simulink model "vehicle_dynamic_dis"  (R2022b)
settings: Solver=VariableStepAuto  StartTime=0.0  StopTime=30  RelTol=1e-3
values from neighbouring files (symbols this model uses):
  A_dis = V_DIS.A    [vehicle_lateral_control_LMIs_3states_auto.m]
  B_dis = V_DIS.B    [vehicle_lateral_control_LMIs_3states_auto.m]
  C_dis = V_DIS.C    [vehicle_lateral_control_LMIs_3states_auto.m]
  D_dis = V_DIS.D    [vehicle_lateral_control_LMIs_3states_auto.m]
  K_gain = K_lmi    [vehicle_lateral_control_LMIs_3states_auto.m]
  Ts = 0.01    [vehicle_lateral_control_LMIs_3states_auto.m]
  vx = 14    [vehicle_lateral_control_LMIs_3states_auto.m]
libraries: cstblocks x1
settings Model: Creator=phatdo  LastModifiedBy=phatdo
settings DataIOCC: ReturnWorkspaceOutputs=off

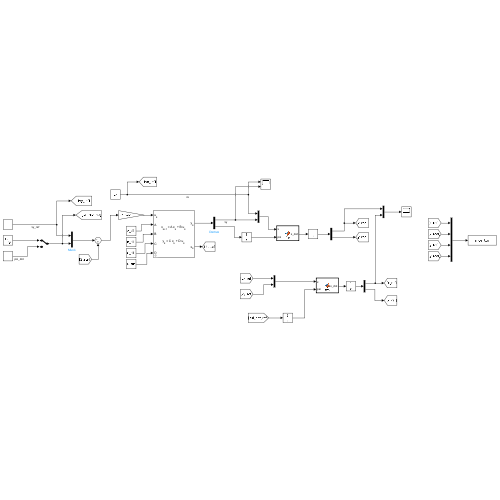
[thumbnail: Simulink's stored preview of the top-level diagram]
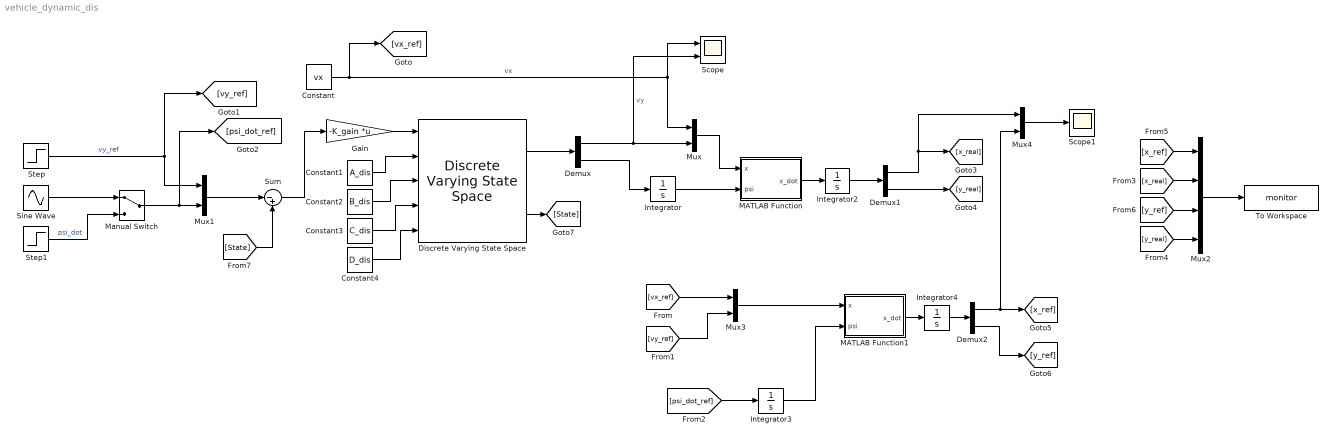
== system vehicle_dynamic_dis ==
  Constant : Constant  Value=vx
  Constant1 : Constant  Value=A_dis
  Constant2 : Constant  Value=B_dis
  Constant3 : Constant  Value=C_dis
  Constant4 : Constant  Value=D_dis
  Demux : Demux  Outputs=2
  Demux1 : Demux  Outputs=2
  Demux2 : Demux  Outputs=2
  Discrete Varying State Space : cstblocks/Linear Parameter Varying/Discrete Varying State Space  x0=0  Ts=Ts  OutputX=on  OutputDX=off
  Gain : Gain  Gain=-K_gain  Multiplication=Matrix(K*u) (u vector)
  Integrator{,2..4} (4 alike) : Integrator
  MATLAB Function : MATLAB Function  TreatAsAtomicUnit=on
  MATLAB Function1 : MATLAB Function  TreatAsAtomicUnit=on
  Manual Switch : ManualSwitch
  Mux{,1,3..4} (4 alike) : Mux  Inputs=2
  Mux2 : Mux
  Scope : Scope  NumInputPorts=2
  Scope1 : Scope
  Sine Wave : Sin  SampleTime=Ts
  Step : Step  Time=0  After=0  SampleTime=Ts
  Step1 : Step  Time=0  After=0.5  SampleTime=Ts
  Sum : Sum  Inputs=|-+
  To Workspace : ToWorkspace  VariableName=monitor  SaveFormat=Timeseries  SampleTime=-1
  wires:
  Discrete Varying State Space/1 -> Demux/1
  Constant/1 -> [vx_ref], Scope/1, Mux/1  "vx"
  Demux/1 -> Scope/2, Mux/2  "vy"
  Mux/1 -> MATLAB Function/1(x)
  Demux/2 -> Integrator/1
  Integrator/1 -> MATLAB Function/2(psi)
  MATLAB Function/1(x_dot) -> Integrator2/1
  Integrator2/1 -> Demux1/1
  Gain/1 -> Discrete Varying State Space/1
  Sum/1 -> Gain/1
  Mux1/1 -> Sum/1
  Step/1 -> [vy_ref], Mux1/1  "vy_ref"
  [psi_dot_ref] -> Integrator3/1
  [vy_ref] -> Mux3/2
  Mux3/1 -> MATLAB Function1/1(x)
  MATLAB Function1/1(x_dot) -> Integrator4/1
  Integrator4/1 -> Demux2/1
  [vx_ref] -> Mux3/1
  Integrator3/1 -> MATLAB Function1/2(psi)
  Demux1/1 -> [x_real], Mux4/1
  Demux1/2 -> [y_real]
  Demux2/1 -> Mux4/2, [x_ref]
  Demux2/2 -> [y_ref]
  [x_ref] -> Mux2/1
  [x_real] -> Mux2/2
  [y_ref] -> Mux2/3
  [y_real] -> Mux2/4
  Mux2/1 -> To Workspace/1
  Mux4/1 -> Scope1/1
  Step1/1 -> Manual Switch/2  "psi_dot"
  Manual Switch/1 -> Mux1/2, [psi_dot_ref]
  Sine Wave/1 -> Manual Switch/1
  Constant1/1 -> Discrete Varying State Space/2
  Constant2/1 -> Discrete Varying State Space/3
  Constant3/1 -> Discrete Varying State Space/4
  Constant4/1 -> Discrete Varying State Space/5
  Discrete Varying State Space/2 -> [State]
  [State] -> Sum/2

== matlab function vehicle_dynamic_dis/MATLAB Function1 ==
  data: x input; x_dot output; psi input
function x_dot = fcn(x, psi)

% x = [vx, vy]

x_dot = zeros(2,1);

vx = x(1);
vy = x(2);

x_dot(1) = vx*cos(psi) - vy*sin(psi);
x_dot(2) = vx*sin(psi) + vy*cos(psi);

end

== matlab function vehicle_dynamic_dis/MATLAB Function ==
  data: x input; x_dot output; psi input
function x_dot = fcn(x, psi)

% x = [vx, vy]

x_dot = zeros(2,1);

vx = x(1);
vy = x(2);

x_dot(1) = vx*cos(psi) - vy*sin(psi);
x_dot(2) = vx*sin(psi) + vy*cos(psi);

end
